simulink model "mix"  (R2024a)
settings: Solver=ode4  StartTime=0.0  StopTime=10.0  FixedStep=0.001  RelTol=1e-3
settings Model: Creator=xiaomi  LastModifiedBy=xiaomi

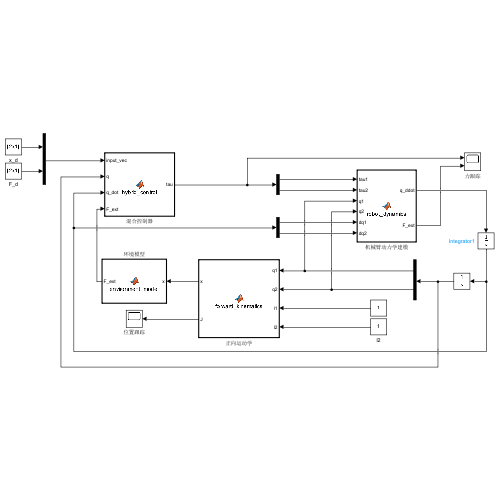
[thumbnail: Simulink's stored preview of the top-level diagram]
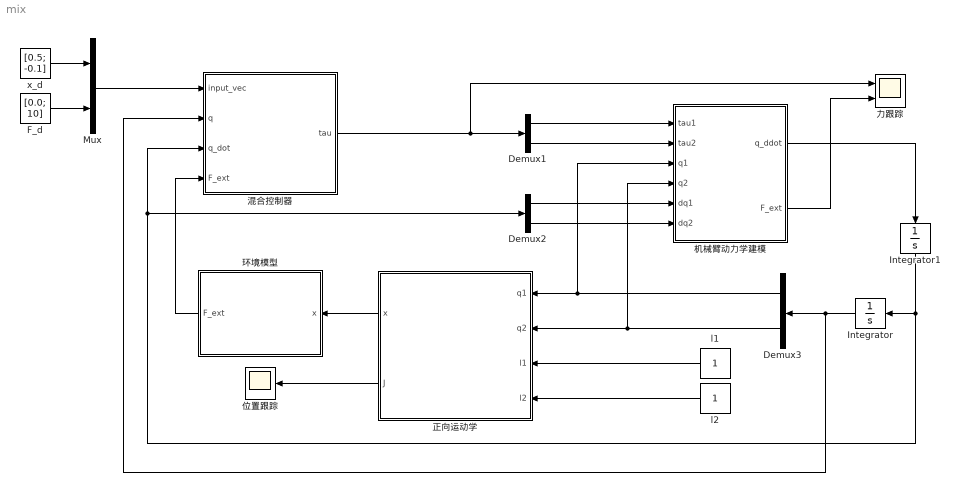
== system mix ==
  Demux1 : Demux  Outputs=2
  Demux2 : Demux  Outputs=2
  Demux3 : Demux  Outputs=2
  F_d : Constant  Value=[0.0; 10]
  Integrator : Integrator  InitialCondition=[0; 0]
  Integrator1 : Integrator  InitialCondition=[0; 0]
  Mux : Mux  Inputs=2
  l1 : Constant
  l2 : Constant
  x_d : Constant  Value=[0.5; -0.1]
  位置跟踪 : Scope
  力跟踪 : Scope  NumInputPorts=2
  机械臂动力学建模 : MATLAB Function  TreatAsAtomicUnit=on
  正向运动学 : MATLAB Function  TreatAsAtomicUnit=on
  混合控制器 : MATLAB Function  TreatAsAtomicUnit=on
  环境模型 : MATLAB Function  TreatAsAtomicUnit=on
  wires:
  x_d/1 -> Mux/1
  F_d/1 -> Mux/2
  Mux/1 -> 混合控制器/1(input_vec)
  Demux1/1 -> 机械臂动力学建模/1(tau1)
  环境模型/1(F_ext) -> 混合控制器/4(F_ext)
  混合控制器/1(tau) -> Demux1/1, 力跟踪/1
  Demux1/2 -> 机械臂动力学建模/2(tau2)
  Demux3/1 -> 机械臂动力学建模/3(q1), 正向运动学/1(q1)
  Demux3/2 -> 机械臂动力学建模/4(q2), 正向运动学/2(q2)
  机械臂动力学建模/1(q_ddot) -> Integrator1/1
  Integrator/1 -> 混合控制器/2(q), Demux3/1
  正向运动学/1(x) -> 环境模型/1(x)
  机械臂动力学建模/2(F_ext) -> 力跟踪/2
  l1/1 -> 正向运动学/3(l1)
  l2/1 -> 正向运动学/4(l2)
  Demux2/1 -> 机械臂动力学建模/5(dq1)
  Demux2/2 -> 机械臂动力学建模/6(dq2)
  Integrator1/1 -> 混合控制器/3(q_dot), Demux2/1, Integrator/1
  正向运动学/2(J) -> 位置跟踪/1

== matlab function mix/机械臂动力学建模 ==
  settings: updateMethod=DISCRETE  sampleTime=0.001
  data: tau1 input; q_ddot output double [0..]; tau2 input; q1 input; q2 input; dq1 input; dq2 input; F_ext output double
function [q_ddot, F_ext] = robot_dynamics(tau1, tau2, q1, q2, dq1, dq2)
% 显式定义所有参数
l1 = 1.0; l2 = 1.0;      % 长度 (m)
m1 = 1.0; m2 = 1.0;      % 质量 (kg)
lc1 = 0.5; lc2 = 0.5;    % 质心位置 (m)
I1 = 0.1; I2 = 0.1;      % 转动惯量
g = 9.81;                % 重力加速度

% ====== 固定大小输出声明 ======
q_ddot = zeros(2, 1);  % 固定2×1向量
F_ext = zeros(2, 1);   % 固定2×1向量

% ====== 惯性矩阵 ======
M11 = m1*lc1^2 + m2*(l1^2 + lc2^2 + 2*l1*lc2*cos(q2)) + I1 + I2;
M12 = m2*(lc2^2 + l1*lc2*cos(q2)) + I2;
M21 = M12;
M22 = m2*lc2^2 + I2;
M = [M11, M12; M21, M22];

% ====== 科里奥利矩阵 ======
c11 = -m2*l1*lc2*sin(q2)*dq2;
c12 = -m2*l1*lc2*sin(q2)*(dq1 + dq2);
c21 = m2*l1*lc2*sin(q2)*dq1;
c22 = 0;
C = [c11, c12; c21, c22];

% ====== 重力项 ======
g1 = (m1*lc1 + m2*l1)*g*cos(q1) + m2*lc2*g*cos(q1+q2);
g2 = m2*lc2*g*cos(q1+q2);
G = [g1; g2];

% ====== 环境接触力 ======
% 内联正运动学
[x, ~] = local_forward_kinematics(q1, q2, l1, l2);
F_ext = local_environment_model(x);

% ====== 动力学方程 ======
tau = [tau1; tau2];
q_dot_vec = [dq1; dq2];
q_ddot = M \ (tau - C*q_dot_vec - G);

% ====== 内联子函数 ======
function [x, J] = local_forward_kinematics(q1, q2, l1, l2)
    x = zeros(2, 1);
    J = zeros(2, 2);
    % 末端位置
    x(1) = l1*cos(q1) + l2*cos(q1+q2);
    x(2) = l1*sin(q1) + l2*sin(q1+q2);
    
    % 雅可比矩阵
    J(1,1) = -l1*sin(q1) - l2*sin(q1+q2);
    J(1,2) = -l2*sin(q1+q2);
    J(2,1) = l1*cos(q1) + l2*cos(q1+q2);
    J(2,2) = l2*cos(q1+q2);
end

function F_ext = local_environment_model(x)
    F_ext = zeros(2, 1);
    surface_y = 0;    % 接触面位置
    K_env = 1500;     % 环境刚度
    D_env = 50;       % 环境阻尼
    mu_k = 0.2;       % 摩擦系数
    
    persistent prev_y;
    if isempty(prev_y)
        prev_y = x(2);
    end
    
    penetration = max(0, surface_y - x(2));
    
    if penetration > 0
        dy_dt = (x(2) - prev_y) / 0.001;
        prev_y = x(2);
        F_y = K_env * penetration + D_env * (-dy_dt);
        F_x = -mu_k * F_y * sign(x(1));
        F_ext(1) = F_x;
        F_ext(2) = F_y;
    else
        F_ext(1) = 0;
        F_ext(2) = 0;
    end
end
end

== matlab function mix/混合控制器 ==
  settings: updateMethod=DISCRETE  sampleTime=0.001
  data: input_vec input; tau output; q input; q_dot input; F_ext input double
function tau = hybrid_control(input_vec, q, q_dot, F_ext)
% 输入: 
%   input_vec = [x_d; F_d] (4×1)
%   q = [q1; q2] (2×1)
%   q_dot = [dq1; dq2] (2×1)
%   F_ext = [F_ext_x; F_ext_y] (2×1)
% 输出: 
%   tau = [tau1; tau2] (2×1)

% ====== 显式定义所有参数 ======
l1 = 1.0;  % 连杆1长度 (m)
l2 = 1.0;  % 连杆2长度 (m)
m1 = 1.0;  % 连杆1质量 (kg)
m2 = 1.0;  % 连杆2质量 (kg)
lc1 = 0.5; % 连杆1质心位置 (m)
lc2 = 0.5; % 连杆2质心位置 (m)
g = 9.81;  % 重力加速度 (m/s²)

% 控制器增益
tau = zeros(2, 1);        % 输出端口初始化
x = zeros(2, 1);          % 位置向量
x_dot = zeros(2, 1);      % 速度向量
e_x = zeros(2, 1);        % 位置误差
e_v = zeros(2, 1);        % 速度误差

% ====== 控制器增益 ======
% 使用显式2×2矩阵代替diag()
Kp = [200, 0; 
       0, 0];   % 位置增益矩阵
Kd = [20, 0;
       0, 0];    % 速度阻尼矩阵
Kfp = 0.8;       % 力比例增益
Kfi = 5.0;       % 力积分增益

% ====== 输入解析 ======
x_d = input_vec(1:2); 
F_d = input_vec(3:4); 

% ====== 运动学计算 ======
[x, J] = forward_kinematics(q(1), q(2), l1, l2);
x_dot = J * q_dot;

% ====== 投影矩阵 ======
n = [0; 1]; 
P_f = n * n';
P_p = eye(2) - P_f;

% ====== 位置控制 ======
e_x = x_d - x;
e_v = -x_dot; 
F_p = P_p * (Kp * e_x + Kd * e_v);

% ====== 力控制 ======
persistent F_integral;
if isempty(F_integral)
    F_integral = [0; 0];  % 确保首次调用时初始化
end

e_F = F_d - F_ext;
F_integral = F_integral + e_F * 0.001;  % dt=0.001s
F_f = P_f * (Kfp * e_F + Kfi * F_integral);

% ====== 动力学补偿 ======
% 内联科里奥利/重力计算
q1 = q(1); q2 = q(2);
dq1 = q_dot(1); dq2 = q_dot(2);

% 科里奥利矩阵
c11 = -m2*l1*lc2*sin(q2)*dq2;
c12 = -m2*l1*lc2*sin(q2)*(dq1 + dq2);
c21 = m2*l1*lc2*sin(q2)*dq1;
c22 = 0;
C = [c11, c12; c21, c22];

% 重力项
g1 = (m1*lc1 + m2*l1)*g*cos(q1) + m2*lc2*g*cos(q1+q2);
g2 = m2*lc2*g*cos(q1+q2);
G = [g1; g2];

% 任务空间转换
J_inv = pinv(J);
C_x = J_inv' * C * J_inv;
G_x = J_inv' * G;

% ====== 总控制力 ======
F_ctrl = F_p + F_f + C_x * x_dot + G_x;
tau = J' * F_ctrl;

% ====== 内联正运动学子函数 ======
function [x, J] = forward_kinematics(q1, q2, l1, l2)
    x = [l1*cos(q1) + l2*cos(q1+q2);
         l1*sin(q1) + l2*sin(q1+q2)];
    
    J11 = -l1*sin(q1) - l2*sin(q1+q2);
    J12 = -l2*sin(q1+q2);
    J21 = l1*cos(q1) + l2*cos(q1+q2);
    J22 = l2*cos(q1+q2);
    J = [J11, J12;
         J21, J22];
end
end

== matlab function mix/环境模型 ==
  settings: updateMethod=DISCRETE  sampleTime=0.001
  data: x input; F_ext output
function F_ext = environment_model(x)
% 模拟 y=0 水平表面接触模型
F_ext = zeros(2,1);  % 添加这一行

surface_y = 0;
K_env = 1500;
D_env = 50;
mu_k = 0.2;

persistent prev_y;
if isempty(prev_y)
    prev_y = x(2);
end

penetration = max(0, surface_y - x(2));
dy_dt = (x(2) - prev_y) / 0.001;
prev_y = x(2);

if penetration > 0
    F_y = K_env * penetration - D_env * dy_dt;
    F_x = -mu_k * F_y * sign(x(1));
else
    F_y = 0;
    F_x = 0;
end

F_ext = [F_x; F_y];
end

== matlab function mix/正向运动学 ==
  settings: updateMethod=DISCRETE  sampleTime=0.001
  data: q1 input; x output; q2 input; l1 input; l2 input; J output
function [x, J] = forward_kinematics(q1, q2, l1, l2) % 添加l1,l2输入
% 末端位置
x = [l1*cos(q1) + l2*cos(q1+q2);
     l1*sin(q1) + l2*sin(q1+q2)];

% 雅可比矩阵
J11 = -l1*sin(q1) - l2*sin(q1+q2);
J12 = -l2*sin(q1+q2);
J21 = l1*cos(q1) + l2*cos(q1+q2);
J22 = l2*cos(q1+q2);
J = [J11, J12;
     J21, J22];
end
